simulink model "fsm"  (R2016b)
settings: Solver=VariableStepAuto  StartTime=0.0  StopTime=10.0  RelTol=1e-3
settings Model: Creator=nadeen  LastModifiedBy=nadeen

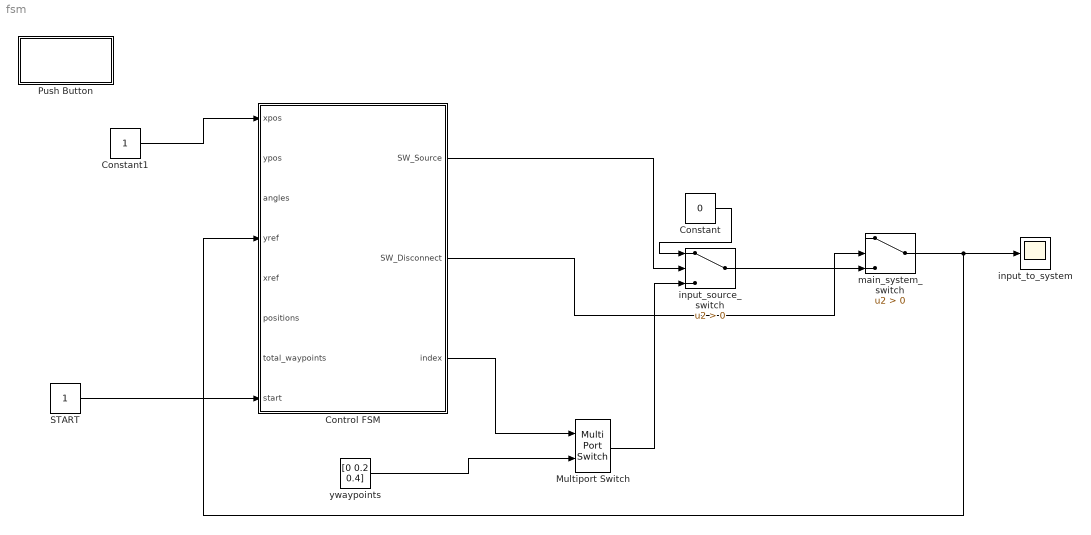
== system fsm ==
  Constant : Constant  Value=0
  Constant1 : Constant
  "Control FSM " : Stateflow chart  TreatAsAtomicUnit=on
  Multiport Switch : MultiPortSwitch  Inputs=1
  Push Button : Subsystem  DialogController=hmiCreateDDGDialog  IsWebBlock=on  mask(MWDashboardBlock){webBlockId=a7d08e25-3ea0-4b4e-9f79-40346c33e361, webBlockType=pushbutton, ShowInLibBrwoser=on, ShowInitialText=on, HMISrcModelName=fsm}
      mask prompts: webBlockId "WebBlock Id"; webBlockType "WebBlock Type"; HMISrcModelName "Source Model"
      mask help: SimulinkHMI:dialogs:PushButtonDialogDesc
      mask Help: helpview([docroot '/mapfiles/simulink.map'], 'hmi_push_button')
      mask Display:
      | model = bdroot(gcb);
      | if strcmp(get_param(model,'BlockDiagramType'), 'library')
      |     image([(matlabroot) '/toolbox/simulink/hmi/icons/PushButton.png']);
      | end
  START : Constant
  input_source_switch : Switch  Criteria=u2 > Threshold
  input_to_system : Scope
  main_system_switch : Switch  Criteria=u2 > Threshold
  ywaypoints : Constant  Value=[0 0.2 0.4]
  wires:
  "Control FSM "/1(SW_Source) -> input_source_switch/2
  "Control FSM "/2(SW_Disconnect) -> main_system_switch/2
  "Control FSM "/3(index) -> Multiport Switch/1
  START/1 -> "Control FSM "/8(start)
  ywaypoints/1 -> Multiport Switch/2
  Constant/1 -> input_source_switch/1
  Multiport Switch/1 -> input_source_switch/3
  input_source_switch/1 -> main_system_switch/3
  main_system_switch/1 -> "Control FSM "/4(yref), input_to_system/1
  Constant1/1 -> "Control FSM "/1(xpos)

== system fsm/Push Button ==

== stateflow chart fsm/Control FSM  ==
  state func1_init(x,y) [function]
    (default) -> (junction 54) : % checks if at 00
    (junction 54) -> (junction 55) [order 1] : [x==0 && y==0]
    (junction 54) -> (junction 56) [order 2] : {ready=0;}
    (junction 55) -> (junction 57) : {ready=1;}
    (junction 57) -> (junction 56)
    (junction 56) -> (junction 58)
  state func2_index_check(i,n) [function]
    (default) -> (junction 73)
    (junction 73) -> (junction 74) [order 1] : [i<=n]
    (junction 73) -> (junction 75) [order 2] : {done=1;}
    (junction 74) -> (junction 76) : { done=0;}
    (junction 76) -> (junction 75)
    (junction 75) -> (junction 77)
  state Idle
    entry:SW_Source=0;
    SW_Disconnect=1;
  state S0_init
    entry: SW_Disconnect=0;
    during:func1_init(xpos,ypos)
    exit: index=1;
  state func3_arrival_check(x,y,xref,yref) [function]
    (default) -> (junction 114)
  state S6_Unstable
    entry:SW_Disconnect=1;
    during:func5_stability_check(angles)
  state func4_problem_check(angles,positions) [function]
    (default) -> (junction 121)
  state S1_index_check
    during:func4_problem_check(angles,positions)
    during:func2_index_check(index,total_waypoints);
  state S7_Resume
    entry:SW_Disconnect=0;
  state S3_increment_index
    entry:index=index+1;
    during:func4_problem_check(angles,positions)
  state S5_Done
    during:func3_arrival_check(xpos,ypos,xref,yref)
  state S4_Moving
    during:func4_problem_check(angles,positions)
    during:func3_arrival_check(xpos,ypos,xref,yref)
  Idle -> S0_init : [start==1]
  (default) -> Idle
  S0_init -> S1_index_check : [ready==1]
  S6_Unstable -> S7_Resume : [stabilized==1]
  S4_Moving -> S6_Unstable [order 2] : [problem==1]
  S3_increment_index -> S6_Unstable [order 2] : [problem==1]
  S4_Moving -> S1_index_check [order 1] : [problem==0 && arrived==1]
  S1_index_check -> S5_Done [order 2] : [done==1]
  S1_index_check -> S3_increment_index [order 1] : [done==0]
  S7_Resume -> S4_Moving
  S3_increment_index -> S4_Moving [order 1] : [problem==0]
  data: x function_input; y function_input; i function_input; n function_input; x function_input; y function_input; xref function_input; yref function_input; angles function_input; positions function_input; xpos input; SW_Source output; SW_Disconnect output; index output; ready local; done local; ypos input; angles input; yref input; xref input; positions input; total_waypoints input; start input; stabilized1 local boolean size=1
